simulink library "sun_point_lib"  (R2016b)
settings: Solver=VariableStepAuto  StartTime=0.0  StopTime=10.0  RelTol=1e-3
undefined symbols (not defined in the file or in its folder): fsw_params
libraries: dspmathops x3, simulink x2, aerolibutil x1
settings Model: Creator=Krish  LastModifiedBy=Taylor

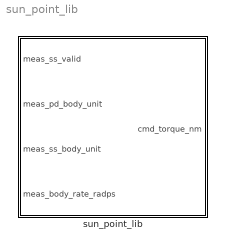
== system sun_point_lib ==
  sun_point_lib : Subsystem  TreatAsAtomicUnit=on
      settings: MinAlgLoopOccurrences=on  RTWFcnNameOpts=Use subsystem name  RTWFileNameOpts=Use subsystem name

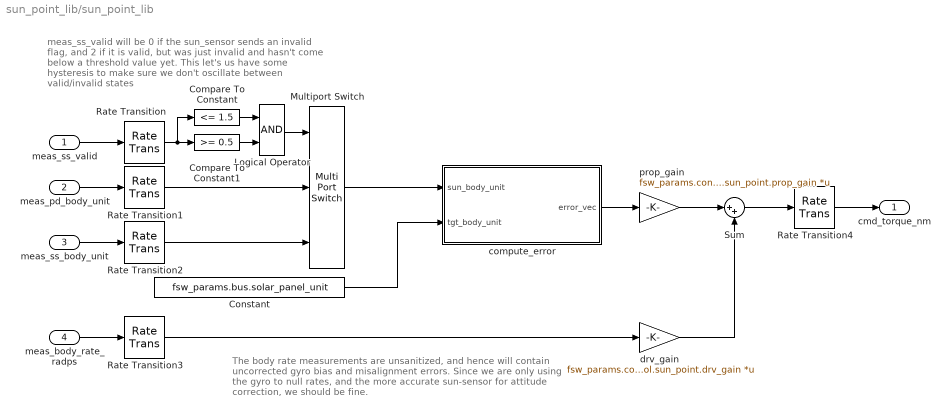
== system sun_point_lib/sun_point_lib ==
  note: meas_ss_valid will be 0 if the sun_sensor sends an
      | invalid flag, and 2 if it is valid, but was just
      | invalid and hasn't come below a threshold value yet.
      | This let's us have some hysteresis to make sure we don't
      | oscillate between valid/invalid states
  note: The body rate measurements are unsanitized, and hence will contain
      | uncorrected gyro bias and misalignment errors. Since we are only using
      | the gyro to null rates, and the more accurate sun-sensor for attitude
      | correction, we should be fine.
  meas_ss_valid : Inport
  meas_pd_body_unit : Inport  Port=2
  meas_ss_body_unit : Inport  Port=3
  meas_body_rate_radps : Inport  Port=4
  Compare To Constant : simulink/Logic and Bit Operations/Compare To Constant  relop=<=  const=1.5  OutDataTypeStr=boolean
  Compare To Constant1 : simulink/Logic and Bit Operations/Compare To Constant  relop=>=  const=0.5  OutDataTypeStr=boolean
  Constant : Constant  Value=fsw_params.bus.solar_panel_unit
  Logical Operator : Logic  AllPortsSameDT=off  OutDataTypeStr=boolean
  Multiport Switch : MultiPortSwitch  DataPortOrder=Zero-based contiguous  Inputs=2
  Rate Transition : RateTransition  X0=fsw_params.control.sun_point.ic.meas_ss_valid  OutPortSampleTime=fsw_params.control.sun_point.sample_time_s
  Rate Transition1 : RateTransition  X0=fsw_params.control.sun_point.ic.meas_pd_body_unit  OutPortSampleTime=fsw_params.control.sun_point.sample_time_s
  Rate Transition2 : RateTransition  X0=fsw_params.control.sun_point.ic.meas_ss_body_unit  OutPortSampleTime=fsw_params.control.sun_point.sample_time_s
  Rate Transition3 : RateTransition  X0=fsw_params.control.sun_point.ic.meas_body_rate_radps  OutPortSampleTime=fsw_params.control.sun_point.sample_time_s
  Rate Transition4 : RateTransition  X0=fsw_params.control.sun_point.ic.cmd_torque_nm  OutPortSampleTimeOpt=Inherit
  Sum : Sum  Inputs=|++
  compute_error : Subsystem
  drv_gain : Gain  Gain=fsw_params.control.sun_point.drv_gain  Multiplication=Matrix(K*u)
  prop_gain : Gain  Gain=fsw_params.control.sun_point.prop_gain  Multiplication=Matrix(K*u)
  cmd_torque_nm : Outport
  wires:
  Multiport Switch/1 -> compute_error/1(sun_body_unit)
  Rate Transition/1 -> Compare To Constant/1, Compare To Constant1/1
  Rate Transition1/1 -> Multiport Switch/2
  Rate Transition3/1 -> drv_gain/1
  meas_pd_body_unit/1 -> Rate Transition1/1
  compute_error/1(error_vec) -> prop_gain/1
  meas_ss_valid/1 -> Rate Transition/1
  Rate Transition2/1 -> Multiport Switch/3
  drv_gain/1 -> Sum/2
  Constant/1 -> compute_error/2(tgt_body_unit)
  meas_ss_body_unit/1 -> Rate Transition2/1
  prop_gain/1 -> Sum/1
  meas_body_rate_radps/1 -> Rate Transition3/1
  Sum/1 -> Rate Transition4/1
  Rate Transition4/1 -> cmd_torque_nm/1
  Compare To Constant/1 -> Logical Operator/1
  Compare To Constant1/1 -> Logical Operator/2
  Logical Operator/1 -> Multiport Switch/1

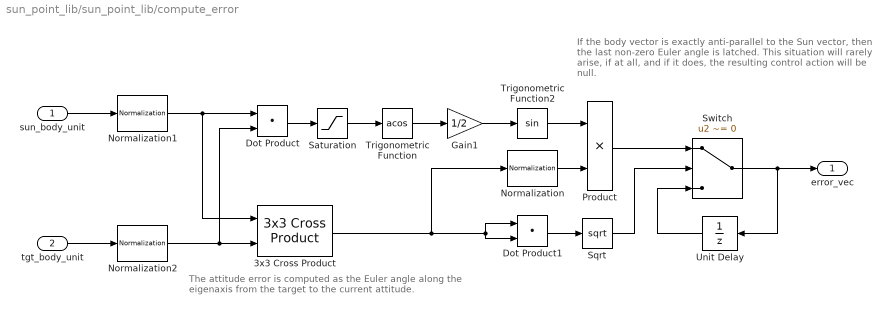
== system sun_point_lib/sun_point_lib/compute_error ==
  note: If the body vector is exactly anti-parallel to the Sun vector,
      | then the last non-zero Euler angle is latched. This situation
      | will rarely arise, if at all, and if it does, the resulting
      | control action will be null.
  note: The attitude error is computed as the Euler angle along the
      | eigenaxis from the target to the current attitude.
  sun_body_unit : Inport
  tgt_body_unit : Inport  Port=2
  3x3 Cross Product : aerolibutil/3x3 Cross Product
  Dot Product : DotProduct  InputSameDT=on  OutDataTypeStr=Inherit: Inherit via internal rule
  Dot Product1 : DotProduct  InputSameDT=on  OutDataTypeStr=Inherit: Inherit via internal rule
  Gain1 : Gain  Gain=1/2
  Normalization : dspmathops/Normalization  NormType=2-norm  Bias=1e-10  NormOver=Each column  Dimension=1  outputDataTypeStr=Inherit: Same as product output  outputLastDataTypeStr=Inherit: Same as product output  outputMin=[]  outputMax=[]  accumDataTypeStr=Inherit: Same as product output  accumLastDataTypeStr=Inherit: Same as product output  roundingMode=Floor  overflowMode=off
  Normalization1 : dspmathops/Normalization  NormType=2-norm  Bias=1e-10  NormOver=Each column  Dimension=1  outputDataTypeStr=Inherit: Same as product output  outputLastDataTypeStr=Inherit: Same as product output  outputMin=[]  outputMax=[]  accumDataTypeStr=Inherit: Same as product output  accumLastDataTypeStr=Inherit: Same as product output  roundingMode=Floor  overflowMode=off
  Normalization2 : dspmathops/Normalization  NormType=2-norm  Bias=1e-10  NormOver=Each column  Dimension=1  outputDataTypeStr=Inherit: Same as product output  outputLastDataTypeStr=Inherit: Same as product output  outputMin=[]  outputMax=[]  accumDataTypeStr=Inherit: Same as product output  accumLastDataTypeStr=Inherit: Same as product output  roundingMode=Floor  overflowMode=off
  Product : Product
  Saturation : Saturate  UpperLimit=1  LowerLimit=-1
      settings: AttributesFormatString=|
      | U: %<UpperLimit>
      | L: %<LowerLimit>
  Sqrt : Sqrt  SaturateOnIntegerOverflow=on
  Switch : Switch  Criteria=u2 ~= 0
  Trigonometric Function : Trigonometry  Operator=acos
  Trigonometric Function2 : Trigonometry
  Unit Delay : UnitDelay  InitialCondition=fsw_params.control.sun_point.ic.error_vec  SampleTime=-1
  error_vec : Outport
  wires:
  tgt_body_unit/1 -> Normalization2/1
  Trigonometric Function2/1 -> Product/1
  Product/1 -> Switch/1
  sun_body_unit/1 -> Normalization1/1
  Saturation/1 -> Trigonometric Function/1
  Gain1/1 -> Trigonometric Function2/1
  Normalization/1 -> Product/2
  Trigonometric Function/1 -> Gain1/1
  Dot Product/1 -> Saturation/1
  Switch/1 -> error_vec/1, Unit Delay/1
  Unit Delay/1 -> Switch/3
  Sqrt/1 -> Switch/2
  Dot Product1/1 -> Sqrt/1
  3x3 Cross Product/1 -> Dot Product1/2, Dot Product1/1, Normalization/1
  Normalization1/1 -> 3x3 Cross Product/1, Dot Product/1
  Normalization2/1 -> Dot Product/2, 3x3 Cross Product/2
